simulink model "HalfCarModel"  (R2022b)
settings: Solver=VariableStepAuto  StartTime=0.0  StopTime=40.0  FixedStep=1e-3  MaxStep=0.01  RelTol=1e-4
undefined symbols (not defined in the file or in its folder): car, f_damper_curve_x, f_damper_curve_y, f_spring_curve_x, f_spring_curve_y, r_damper_curve_x, r_damper_curve_y, r_spring_curve_x, r_spring_curve_y
settings Model: Creator=Louis  LastModifiedBy=Louis
settings DebuggingCC: AlgebraicLoopMsg=none  UnderspecifiedInitializationDetection=Classic  MergeDetectMultiDrivingBlocksExec=none
settings ModelReferenceCC: PropagateSignalLabelsOutOfModel=off

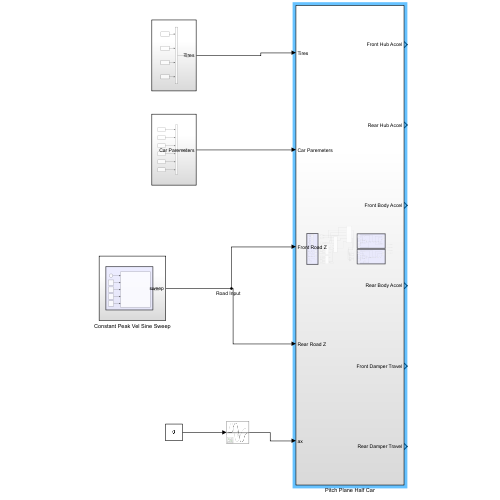
[thumbnail: Simulink's stored preview of the top-level diagram]
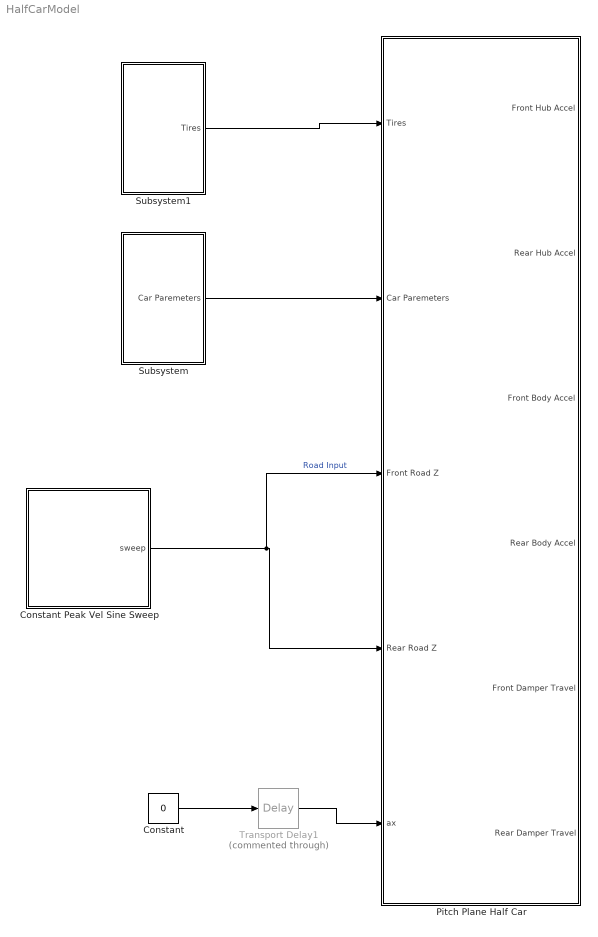
== system HalfCarModel ==
  Constant : Constant  Value=0
  Constant Peak Vel Sine Sweep : Subsystem
  Pitch Plane Half Car : Subsystem
  Subsystem : Subsystem
  Subsystem1 : Subsystem
  Transport Delay1 : TransportDelay  Commented=through  DelayTime=3
  wires:
  Constant/1 -> Transport Delay1/1
  Subsystem/1(Car Paremeters) -> Pitch Plane Half Car/2(Car Paremeters)
  Subsystem1/1(Tires) -> Pitch Plane Half Car/1(Tires)
  Constant Peak Vel Sine Sweep/1(sweep) -> Pitch Plane Half Car/4(Rear Road Z), Pitch Plane Half Car/3(Front Road Z)  "Road Input"
  Transport Delay1/1 -> Pitch Plane Half Car/5(ax)

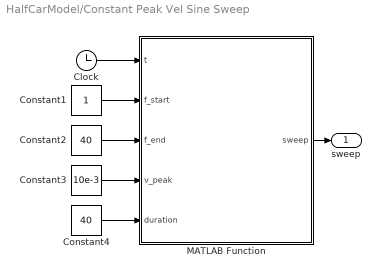
== system HalfCarModel/Constant Peak Vel Sine Sweep ==
  Clock : Clock
  Constant1 : Constant
  Constant2 : Constant  Value=40
  Constant3 : Constant  Value=10e-3
  Constant4 : Constant  Value=40
  MATLAB Function : MATLAB Function  TreatAsAtomicUnit=on
  sweep : Outport
  wires:
  Constant3/1 -> MATLAB Function/4(v_peak)
  MATLAB Function/1(sweep) -> sweep/1
  Constant4/1 -> MATLAB Function/5(duration)
  Clock/1 -> MATLAB Function/1(t)
  Constant2/1 -> MATLAB Function/3(f_end)
  Constant1/1 -> MATLAB Function/2(f_start)

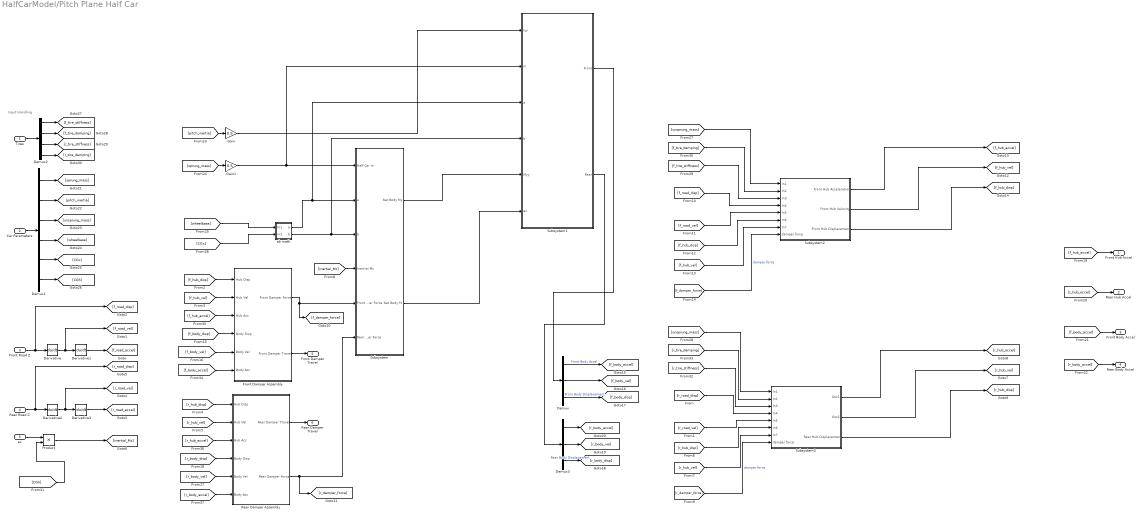
== system HalfCarModel/Pitch Plane Half Car ==
  note: Input Handling
  Tires : Inport
  Car Paremeters : Inport  Port=2
  Front Road Z : Inport  Port=3
  Rear Road Z : Inport  Port=4
  ax : Inport  Port=5
  Demux : Demux  Outputs=3
  Demux1 : Demux  Outputs=6
  Demux2 : Demux
  Demux3 : Demux  Outputs=3
  Derivative{,1..3} (4 alike) : Derivative
  Front Damper Assembly : Subsystem
  Gain : Gain  Gain=0.5
  Gain1 : Gain  Gain=0.5
  Product : Product
  Rear Damper Assembly : Subsystem
  Subsystem : Subsystem
  Subsystem1 : Subsystem
  Subsystem2 : Subsystem
  Subsystem3 : Subsystem
  ab math : Subsystem
  Front Hub Accel : Outport
  Rear Hub Accel : Outport  Port=2
  Front Body Accel : Outport  Port=3
  Rear Body Accel : Outport  Port=4
  Front Damper Travel : Outport  Port=5
  Rear Damper Travel : Outport  Port=6
  wires:
  Front Road Z/1 -> Derivative/1, [f_road_disp]
  Derivative/1 -> [f_road_vel], Derivative1/1
  Derivative1/1 -> [f_road_accel]
  Derivative2/1 -> [r_road_vel], Derivative3/1
  Rear Road Z/1 -> [r_road_disp], Derivative2/1
  Derivative3/1 -> [r_road_accel]
  ax/1 -> Product/1
  [CGh] -> Product/2
  Product/1 -> [inertial_Mz]
  [f_hub_accel] -> Front Hub Accel/1
  [r_hub_accel] -> Rear Hub Accel/1
  [f_body_accel] -> Front Body Accel/1
  [r_body_accel] -> Rear Body Accel/1
  Car Paremeters/1 -> Demux1/1
  Demux1/1 -> [sprung_mass]
  Demux1/2 -> [pitch_inertia]
  Demux1/3 -> [unsprung_mass]
  Demux1/4 -> [wheelbase]
  Demux1/5 -> [CGx]
  Demux1/6 -> [CGh]
  Tires/1 -> Demux2/1
  Demux2/1 -> [f_tire_stiffness]
  Demux2/2 -> [f_tire_damping]
  Demux2/3 -> [r_tire_stiffness]
  Demux2/4 -> [r_tire_damping]
  Front Damper Assembly/1(Front Damper Force) -> [f_damper_force], Subsystem/5(Front Damper Force)
  [f_hub_disp] -> Front Damper Assembly/1(Hub Disp)
  [f_hub_vel] -> Front Damper Assembly/2(Hub Vel)
  [f_hub_accel] -> Front Damper Assembly/3(Hub Acc)
  [f_body_disp] -> Front Damper Assembly/4(Body Disp)
  [f_body_vel] -> Front Damper Assembly/5(Body Vel)
  [f_body_accel] -> Front Damper Assembly/6(Body Acc)
  Front Damper Assembly/2(Front Damper Travel) -> Front Damper Travel/1
  Rear Damper Assembly/2(Rear Damper Force) -> [r_damper_force], Subsystem/6(Rear Damper Force)
  [r_hub_disp] -> Rear Damper Assembly/1(Hub Disp)
  [r_hub_vel] -> Rear Damper Assembly/2(Hub Vel)
  [r_hub_accel] -> Rear Damper Assembly/3(Hub Acc)
  [r_body_disp] -> Rear Damper Assembly/4(Body Disp)
  [r_body_vel] -> Rear Damper Assembly/5(Body Vel)
  [r_body_accel] -> Rear Damper Assembly/6(Body Acc)
  Rear Damper Assembly/1(Rear Damper Travel) -> Rear Damper Travel/1
  [inertial_Mz] -> Subsystem/4(Inertial Mz)
  [pitch_inertia] -> Gain/1
  [sprung_mass] -> Gain1/1
  Gain1/1 -> Subsystem/1(Half Car m), Subsystem1/2(m)
  [wheelbase] -> ab math/1(In1)
  [CGx] -> ab math/2(In2)
  ab math/1(a) -> Subsystem/2(a), Subsystem1/3(a)
  ab math/2(b) -> Subsystem/3(b), Subsystem1/4(b)
  Gain/1 -> Subsystem1/1(Iyy)
  Subsystem/1(Net Body My) -> Subsystem1/5(Myy)
  Subsystem/2(Net Body Fz) -> Subsystem1/6(az)
  Demux/1 -> [f_body_accel]  "Front Body Accel"
  Demux/2 -> [f_body_vel]
  Demux/3 -> [f_body_disp]  "Front Body Displacement"
  Demux3/2 -> [r_body_vel]
  Demux3/3 -> [r_body_disp]  "Rear Body Displacement"
  Demux3/1 -> [r_body_accel]
  Subsystem1/1(Front) -> Demux/1
  Subsystem1/2(Rear) -> Demux3/1
  [unsprung_mass] -> Subsystem2/1(In1)
  [f_tire_damping] -> Subsystem2/2(In2)
  [f_tire_stiffness] -> Subsystem2/3(In3)
  [f_road_disp] -> Subsystem2/4(In4)
  [f_road_vel] -> Subsystem2/5(In5)
  [f_hub_disp] -> Subsystem2/6(In6)
  [f_hub_vel] -> Subsystem2/7(In7)
  [f_damper_force] -> Subsystem2/8(damper force)  "damper force"
  Subsystem2/1(Front Hub Acceleration) -> [f_hub_accel]
  Subsystem2/2(Front Hub Velocity) -> [f_hub_vel]
  Subsystem2/3(Front Hub Displacement) -> [f_hub_disp]
  [unsprung_mass] -> Subsystem3/1(In1)
  [r_tire_damping] -> Subsystem3/2(In2)
  [r_tire_stiffness] -> Subsystem3/3(In3)
  [r_road_disp] -> Subsystem3/4(In4)
  [r_road_vel] -> Subsystem3/5(In5)
  [r_hub_disp] -> Subsystem3/6(In6)
  [r_hub_vel] -> Subsystem3/7(In7)
  [r_damper_force] -> Subsystem3/8(damper force)  "damper force"
  Subsystem3/1(Out1) -> [r_hub_accel]
  Subsystem3/2(Out2) -> [r_hub_vel]
  Subsystem3/3(Rear Hub Displacement) -> [r_hub_disp]

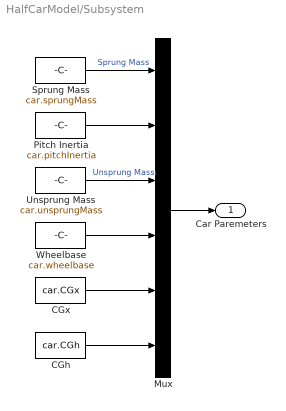
== system HalfCarModel/Subsystem ==
  CGh : Constant  Value=car.CGh
  CGx : Constant  Value=car.CGx
  Mux : Mux  Inputs=6
  Pitch Inertia : Constant  Value=car.pitchInertia
  Sprung Mass : Constant  Value=car.sprungMass
  Unsprung Mass : Constant  Value=car.unsprungMass
  Wheelbase : Constant  Value=car.wheelbase
  Car Paremeters : Outport
  wires:
  Sprung Mass/1 -> Mux/1  "Sprung Mass"
  Wheelbase/1 -> Mux/4
  Pitch Inertia/1 -> Mux/2
  Unsprung Mass/1 -> Mux/3  "Unsprung Mass"
  CGh/1 -> Mux/6
  CGx/1 -> Mux/5
  Mux/1 -> Car Paremeters/1

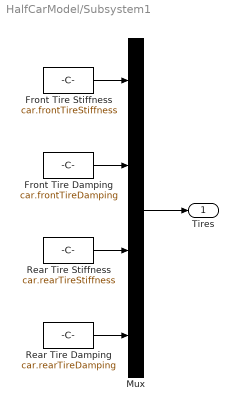
== system HalfCarModel/Subsystem1 ==
  Front Tire Damping : Constant  Value=car.frontTireDamping
  Front Tire Stiffness : Constant  Value=car.frontTireStiffness
  Mux : Mux
  Rear Tire Damping : Constant  Value=car.rearTireDamping
  Rear Tire Stiffness : Constant  Value=car.rearTireStiffness
  Tires : Outport
  wires:
  Mux/1 -> Tires/1
  Rear Tire Stiffness/1 -> Mux/3
  Front Tire Damping/1 -> Mux/2
  Rear Tire Damping/1 -> Mux/4
  Front Tire Stiffness/1 -> Mux/1

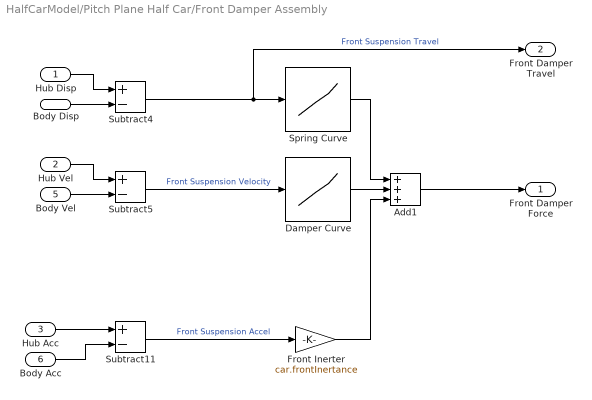
== system HalfCarModel/Pitch Plane Half Car/Front Damper Assembly ==
  Hub Disp : Inport
  Hub Vel : Inport  Port=2
  Hub Acc : Inport  Port=3
  Body Disp : Inport  Port=4
  Body Vel : Inport  Port=5
  Body Acc : Inport  Port=6
  Add1 : Sum  Inputs=+++
  Damper Curve : Lookup_n-D  NumberOfTableDimensions=1  BreakpointsForDimension1=f_damper_curve_x  Table=f_damper_curve_y  InterpMethod=Linear Lagrange  InternalRulePriority=Speed  RndMeth=Simplest
  Front Inerter : Gain  Gain=car.frontInertance
  Spring Curve : Lookup_n-D  NumberOfTableDimensions=1  BreakpointsForDimension1=f_spring_curve_x  Table=f_spring_curve_y  InterpMethod=Linear Lagrange  InternalRulePriority=Speed  RndMeth=Simplest
  Subtract11 : Sum  Inputs=+-
  Subtract4 : Sum  Inputs=+-
  Subtract5 : Sum  Inputs=+-
  Front Damper Force : Outport
  Front Damper Travel : Outport  Port=2
  wires:
  Subtract11/1 -> Front Inerter/1  "Front Suspension Accel"
  Front Inerter/1 -> Add1/3
  Damper Curve/1 -> Add1/2
  Hub Vel/1 -> Subtract5/1
  Subtract4/1 -> Front Damper Travel/1, Spring Curve/1  "Front Suspension Travel"
  Spring Curve/1 -> Add1/1
  Hub Disp/1 -> Subtract4/1
  Subtract5/1 -> Damper Curve/1  "Front Suspension Velocity"
  Add1/1 -> Front Damper Force/1
  Body Disp/1 -> Subtract4/2
  Body Vel/1 -> Subtract5/2
  Body Acc/1 -> Subtract11/2
  Hub Acc/1 -> Subtract11/1

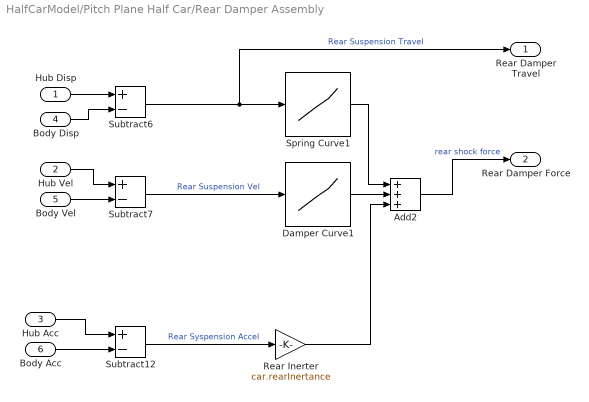
== system HalfCarModel/Pitch Plane Half Car/Rear Damper Assembly ==
  Hub Disp : Inport
  Hub Vel : Inport  Port=2
  Hub Acc : Inport  Port=3
  Body Disp : Inport  Port=4
  Body Vel : Inport  Port=5
  Body Acc : Inport  Port=6
  Add2 : Sum  Inputs=+++
  Damper Curve1 : Lookup_n-D  NumberOfTableDimensions=1  BreakpointsForDimension1=r_damper_curve_x  Table=r_damper_curve_y  InterpMethod=Linear Lagrange  InternalRulePriority=Speed  RndMeth=Simplest
  Rear Inerter : Gain  Gain=car.rearInertance
  Spring Curve1 : Lookup_n-D  NumberOfTableDimensions=1  BreakpointsForDimension1=r_spring_curve_x  Table=r_spring_curve_y  InterpMethod=Linear Lagrange  InternalRulePriority=Speed  RndMeth=Simplest
  Subtract12 : Sum  Inputs=+-
  Subtract6 : Sum  Inputs=+-
  Subtract7 : Sum  Inputs=+-
  Rear Damper Travel : Outport
  Rear Damper Force : Outport  Port=2
  wires:
  Hub Disp/1 -> Subtract6/1
  Damper Curve1/1 -> Add2/2
  Subtract6/1 -> Rear Damper Travel/1, Spring Curve1/1  "Rear Suspension Travel"
  Spring Curve1/1 -> Add2/1
  Hub Vel/1 -> Subtract7/1
  Subtract7/1 -> Damper Curve1/1  "Rear Suspension Vel"
  Subtract12/1 -> Rear Inerter/1  "Rear Syspension Accel"
  Rear Inerter/1 -> Add2/3
  Add2/1 -> Rear Damper Force/1  "rear shock force"
  Body Vel/1 -> Subtract7/2
  Body Disp/1 -> Subtract6/2
  Hub Acc/1 -> Subtract12/1
  Body Acc/1 -> Subtract12/2

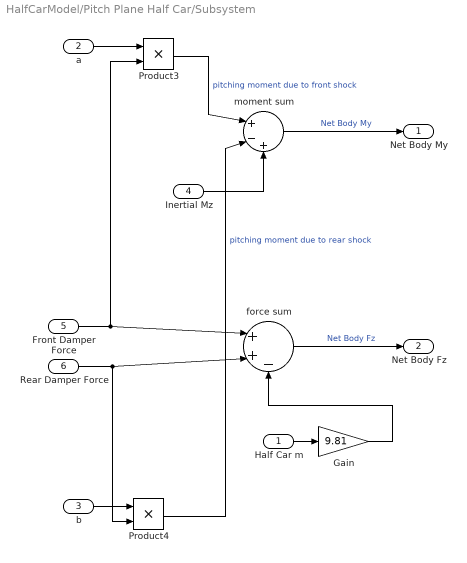
== system HalfCarModel/Pitch Plane Half Car/Subsystem ==
  Half Car m : Inport
  a : Inport  Port=2
  b : Inport  Port=3
  Inertial Mz : Inport  Port=4
  Front Damper Force : Inport  Port=5
  Rear Damper Force : Inport  Port=6
  Gain : Gain  Gain=9.81
  Product3 : Product
  Product4 : Product
  force sum : Sum  Inputs=|++-
  moment sum : Sum  Inputs=|+-+
  Net Body My : Outport
  Net Body Fz : Outport  Port=2
  wires:
  Front Damper Force/1 -> Product3/2, force sum/1
  Product3/1 -> moment sum/1  "pitching moment due to front shock"
  Product4/1 -> moment sum/2  "pitching moment due to rear shock"
  force sum/1 -> Net Body Fz/1  "Net Body Fz"
  Inertial Mz/1 -> moment sum/3
  Rear Damper Force/1 -> Product4/2, force sum/2
  moment sum/1 -> Net Body My/1  "Net Body My"
  Half Car m/1 -> Gain/1
  Gain/1 -> force sum/3
  a/1 -> Product3/1
  b/1 -> Product4/1

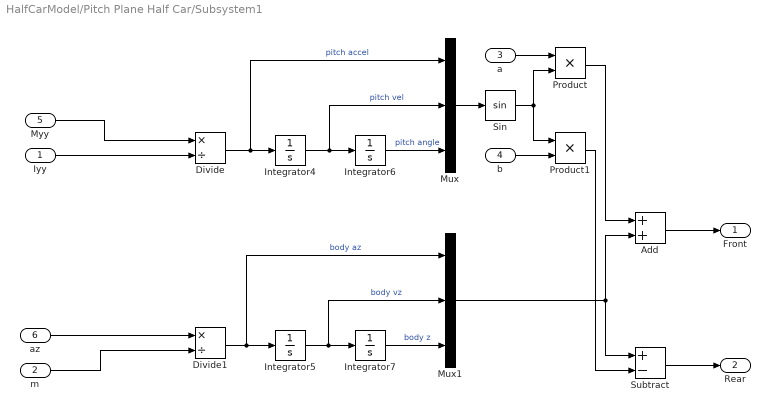
== system HalfCarModel/Pitch Plane Half Car/Subsystem1 ==
  Iyy : Inport
  m : Inport  Port=2
  a : Inport  Port=3
  b : Inport  Port=4
  Myy : Inport  Port=5
  az : Inport  Port=6
  Add : Sum
  Divide : Product  Inputs=*/
  Divide1 : Product  Inputs=*/
  Integrator{4..7} (4 alike) : Integrator
  Mux : Mux  Inputs=3
  Mux1 : Mux  Inputs=3
  Product : Product
  Product1 : Product
  Sin : Trigonometry
  Subtract : Sum  Inputs=+-
  Front : Outport
  Rear : Outport  Port=2
  wires:
  Divide/1 -> Mux/1, Integrator4/1  "pitch accel"
  Divide1/1 -> Mux1/1, Integrator5/1  "body az"
  Integrator4/1 -> Mux/2, Integrator6/1  "pitch vel"
  Iyy/1 -> Divide/2
  Integrator5/1 -> Mux1/2, Integrator7/1  "body vz"
  az/1 -> Divide1/1
  Myy/1 -> Divide/1
  m/1 -> Divide1/2
  Integrator6/1 -> Mux/3  "pitch angle"
  Integrator7/1 -> Mux1/3  "body z"
  Mux/1 -> Sin/1
  Sin/1 -> Product1/1, Product/2
  a/1 -> Product/1
  b/1 -> Product1/2
  Mux1/1 -> Subtract/1, Add/2
  Product/1 -> Add/1
  Product1/1 -> Subtract/2
  Add/1 -> Front/1
  Subtract/1 -> Rear/1

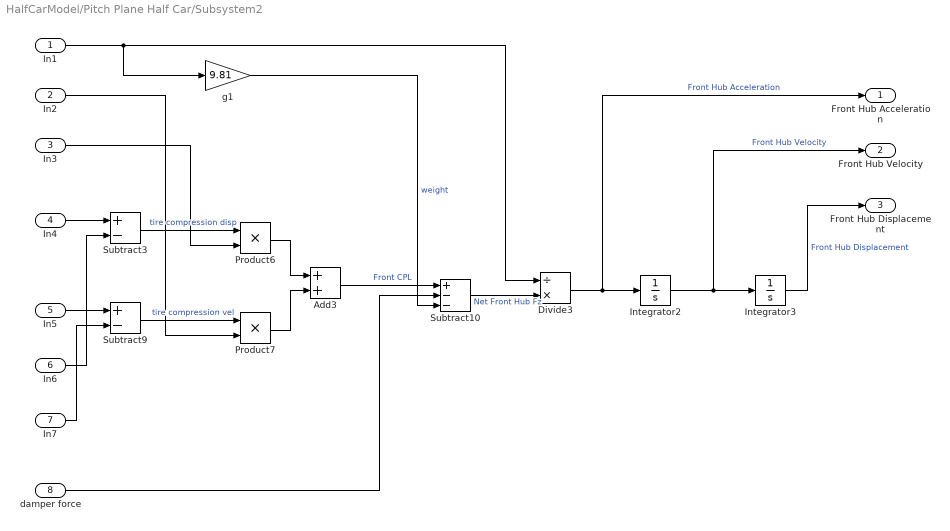
== system HalfCarModel/Pitch Plane Half Car/Subsystem2 ==
  In1 : Inport
  In2 : Inport  Port=2
  In3 : Inport  Port=3
  In4 : Inport  Port=4
  In5 : Inport  Port=5
  In6 : Inport  Port=6
  In7 : Inport  Port=7
  damper force : Inport  Port=8
  Add3 : Sum
  Divide3 : Product  Inputs=/*
  Integrator2 : Integrator
  Integrator3 : Integrator
  Product6 : Product
  Product7 : Product
  Subtract10 : Sum  Inputs=+--
  Subtract3 : Sum  Inputs=+-
  Subtract9 : Sum  Inputs=+-
  g1 : Gain  Gain=9.81
  Front Hub Acceleration : Outport
  Front Hub Velocity : Outport  Port=2
  Front Hub Displacement : Outport  Port=3
  wires:
  Subtract9/1 -> Product7/1  "tire compression vel"
  Product6/1 -> Add3/1
  Subtract10/1 -> Divide3/2  "Net Front Hub Fz"
  Divide3/1 -> Front Hub Acceleration/1, Integrator2/1  "Front Hub Acceleration"
  In1/1 -> Divide3/1, g1/1
  Subtract3/1 -> Product6/1  "tire compression disp"
  Integrator2/1 -> Front Hub Velocity/1, Integrator3/1  "Front Hub Velocity"
  g1/1 -> Subtract10/3  "weight"
  Product7/1 -> Add3/2
  Add3/1 -> Subtract10/1  "Front CPL"
  In5/1 -> Subtract9/1
  In3/1 -> Product6/2
  In4/1 -> Subtract3/1
  In2/1 -> Product7/2
  damper force/1 -> Subtract10/2
  Integrator3/1 -> Front Hub Displacement/1  "Front Hub Displacement"
  In6/1 -> Subtract3/2
  In7/1 -> Subtract9/2

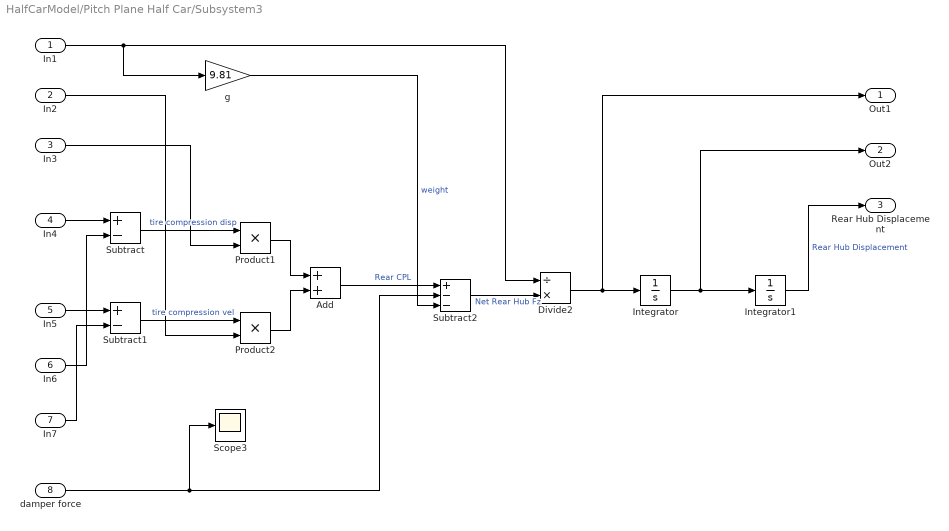
== system HalfCarModel/Pitch Plane Half Car/Subsystem3 ==
  In1 : Inport
  In2 : Inport  Port=2
  In3 : Inport  Port=3
  In4 : Inport  Port=4
  In5 : Inport  Port=5
  In6 : Inport  Port=6
  In7 : Inport  Port=7
  damper force : Inport  Port=8
  Add : Sum
  Divide2 : Product  Inputs=/*
  Integrator : Integrator
  Integrator1 : Integrator
  Product1 : Product
  Product2 : Product
  Scope3 : Scope
  Subtract : Sum  Inputs=+-
  Subtract1 : Sum  Inputs=+-
  Subtract2 : Sum  Inputs=+--
  g : Gain  Gain=9.81
  Out1 : Outport
  Out2 : Outport  Port=2
  Rear Hub Displacement : Outport  Port=3
  wires:
  Subtract2/1 -> Divide2/2  "Net Rear Hub Fz"
  Add/1 -> Subtract2/1  "Rear CPL"
  damper force/1 -> Scope3/1, Subtract2/2
  Subtract1/1 -> Product2/1  "tire compression vel"
  g/1 -> Subtract2/3  "weight"
  Product1/1 -> Add/1
  Product2/1 -> Add/2
  Integrator/1 -> Out2/1, Integrator1/1
  In1/1 -> Divide2/1, g/1
  Subtract/1 -> Product1/1  "tire compression disp"
  Divide2/1 -> Out1/1, Integrator/1
  In6/1 -> Subtract/2
  Integrator1/1 -> Rear Hub Displacement/1  "Rear Hub Displacement"
  In3/1 -> Product1/2
  In4/1 -> Subtract/1
  In7/1 -> Subtract1/2
  In2/1 -> Product2/2
  In5/1 -> Subtract1/1

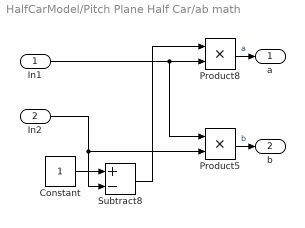
== system HalfCarModel/Pitch Plane Half Car/ab math ==
  In1 : Inport
  In2 : Inport  Port=2
  Constant : Constant
  Product5 : Product
  Product8 : Product
  Subtract8 : Sum  Inputs=+-
  a : Outport
  b : Outport  Port=2
  wires:
  Constant/1 -> Subtract8/1
  Product8/1 -> a/1  "a"
  In1/1 -> Product5/1, Product8/2
  Subtract8/1 -> Product8/1
  In2/1 -> Subtract8/2, Product5/2
  Product5/1 -> b/1  "b"

== matlab function HalfCarModel/Constant Peak Vel Sine Sweep/MATLAB Function ==
  data: t input; f_start input; sweep output; f_end input; v_peak input; duration input
function sweep = sineSweepFunc(t, f_start, f_end, v_peak, duration)
% SINESWEEPFUNC creates a continuous-time sine sweep with constant peak velocity.
% Returns function handles sweep.v(t) and sweep.x(t)
% Modified to include 10-second wait at zero and smooth start

    wait_time = 10.0;  % 10-second wait time at zero
    total_time = wait_time + duration;
    
    % Initialize output with zeros
    sweep = zeros(size(t));
    
    % For times during the wait period
    wait_indices = t < wait_time;
    
    % For times during the sweep period
    sweep_indices = t >= wait_time & t <= total_time;
    
    % During wait period: everything is zero
    sweep(wait_indices) = 0;
    
    % During sweep period: apply modified sine sweep with smooth start
    if any(sweep_indices)
        t_sweep = t(sweep_indices) - wait_time;  % Shift time to start at 0
        
        k = log(f_end / f_start);  % logarithmic rate factor
        
        % Modified phase function with smooth start
        % Add a cosine taper for the first 5% of the sweep to smooth the start
        ramp_fraction = 0.05;
        ramp_time = ramp_fraction * duration;
        
        % Create a smooth ramp-up window
        ramp_window = ones(size(t_sweep));
        ramp_indices = t_sweep < ramp_time;
        if any(ramp_indices)
            % Cosine taper for smooth transition from 0 to 1
            ramp_window(ramp_indices) = 0.5 * (1 - cos(pi * t_sweep(ramp_indices) / ramp_time));
        end
        
        % Phase function φ(t)
        phi = 2*pi*f_start*duration*(exp((k .* t_sweep) ./ duration) - 1) ./ k;
        
        % Frequency at each time instant
        f_instant = f_start * exp((k .* t_sweep) ./ duration);
        
        % Displacement with ramp window applied
        sweep(sweep_indices) = -ramp_window .* v_peak ./ (2*pi*f_instant) .* cos(phi);
    end
    
    % For times after the sweep (hold at final position)
    if max(t) > total_time
        post_indices = t > total_time;
        % Get the final displacement value from the end of sweep
        if any(sweep_indices)
            final_disp = sweep(find(sweep_indices, 1, 'last'));
            sweep(post_indices) = final_disp;
        end
    end
end
